simulink model "VCU_CS75_12_16_Test"  (R2014a)
settings: Solver=FixedStepDiscrete  StartTime=0.0  StopTime=25  FixedStep=0.0005  RelTol=1e-3
undefined symbols (not defined in the file): ecucoder_acal, I_SW01_L, LaterlAngleCommand, LDW, RemoteAcclPosition
libraries: simulink x913, ec5744lib x39
(part 6 of 30)

== system VCU_CS75_12_16_Test/长安CS75底盘程序，20ms一次/Input/DBC转化的messages（存底）/ReceiveMessages18/BCM_328 ==
  input : Inport
  Demux : Demux  Outputs=8
  LCM_DRLSts_Ad : Sum
  LCM_DRLSts_Convert : DataTypeConversion  OutDataTypeStr=uint32
  LCM_DRLSts_F : Gain
  LCM_DRLSts_L : simulink/Logic and Bit Operations/Bitwise Operator  logicop=AND  UseBitMask=on  BitMask=192  BitMaskRealWorld=Stored Integer
  LCM_DRLSts_O : Constant  Value=0  OutDataTypeStr=single
  LCM_DRLSts_S : ArithShift  BitShiftNumber=6
  LCM_DRLSts_Sub : Subsystem
  LCM_DRLSts_sat : Saturate  UpperLimit=0  LowerLimit=0
  LCM_DRLStscv : DataTypeConversion
  LCM_DriveMode_Ad : Sum
  LCM_DriveMode_Convert : DataTypeConversion  OutDataTypeStr=uint32
  LCM_DriveMode_F : Gain
  LCM_DriveMode_L : simulink/Logic and Bit Operations/Bitwise Operator  logicop=AND  UseBitMask=on  BitMask=192  BitMaskRealWorld=Stored Integer
  LCM_DriveMode_O : Constant  Value=0  OutDataTypeStr=single
  LCM_DriveMode_S : ArithShift  BitShiftNumber=6
  LCM_DriveMode_Sub : Subsystem
  LCM_DriveMode_sat : Saturate  UpperLimit=0  LowerLimit=0
  LCM_DriveModecv : DataTypeConversion
  LCM_LASSwitch_Ad : Sum
  LCM_LASSwitch_Convert : DataTypeConversion  OutDataTypeStr=uint32
  LCM_LASSwitch_F : Gain
  LCM_LASSwitch_L : simulink/Logic and Bit Operations/Bitwise Operator  logicop=AND  UseBitMask=on  BitMask=3  BitMaskRealWorld=Stored Integer
  LCM_LASSwitch_O : Constant  Value=0  OutDataTypeStr=single
  LCM_LASSwitch_S : ArithShift
  LCM_LASSwitch_Sub : Subsystem
  LCM_LASSwitch_sat : Saturate  UpperLimit=3  LowerLimit=0
  LCM_LASSwitchcv : DataTypeConversion
  LCM_RearLeftTuningLightFaultSts_Ad : Sum
  LCM_RearLeftTuningLightFaultSts_Convert : DataTypeConversion  OutDataTypeStr=uint32
  LCM_RearLeftTuningLightFaultSts_F : Gain
  LCM_RearLeftTuningLightFaultSts_L : simulink/Logic and Bit Operations/Bitwise Operator  logicop=AND  UseBitMask=on  BitMask=128  BitMaskRealWorld=Stored Integer
  LCM_RearLeftTuningLightFaultSts_O : Constant  Value=0  OutDataTypeStr=single
  LCM_RearLeftTuningLightFaultSts_S : ArithShift  BitShiftNumber=7
  LCM_RearLeftTuningLightFaultSts_Sub : Subsystem
  LCM_RearLeftTuningLightFaultSts_sat : Saturate  UpperLimit=0  LowerLimit=0
  LCM_RearLeftTuningLightFaultStscv : DataTypeConversion
  LCM_RearRightTuningLightFaultSts_Ad : Sum
  LCM_RearRightTuningLightFaultSts_Convert : DataTypeConversion  OutDataTypeStr=uint32
  LCM_RearRightTuningLightFaultSts_F : Gain
  LCM_RearRightTuningLightFaultSts_L : simulink/Logic and Bit Operations/Bitwise Operator  logicop=AND  UseBitMask=on  BitMask=128  BitMaskRealWorld=Stored Integer
  LCM_RearRightTuningLightFaultSts_O : Constant  Value=0  OutDataTypeStr=single
  LCM_RearRightTuningLightFaultSts_S : ArithShift  BitShiftNumber=7
  LCM_RearRightTuningLightFaultSts_Sub : Subsystem
  LCM_RearRightTuningLightFaultSts_sat : Saturate  UpperLimit=0  LowerLimit=0
  LCM_RearRightTuningLightFaultStscv : DataTypeConversion
  LCM_ReverseLightSts_Ad : Sum
  LCM_ReverseLightSts_Convert : DataTypeConversion  OutDataTypeStr=uint32
  LCM_ReverseLightSts_F : Gain
  LCM_ReverseLightSts_L : simulink/Logic and Bit Operations/Bitwise Operator  logicop=AND  UseBitMask=on  BitMask=192  BitMaskRealWorld=Stored Integer
  LCM_ReverseLightSts_O : Constant  Value=0  OutDataTypeStr=single
  LCM_ReverseLightSts_S : ArithShift  BitShiftNumber=6
  LCM_ReverseLightSts_Sub : Subsystem
  LCM_ReverseLightSts_sat : Saturate  UpperLimit=0  LowerLimit=0
  LCM_ReverseLightStscv : DataTypeConversion
  LCM_DriveMode_Out : Outport
  LCM_DRLSts_Out : Outport  Port=2
  LCM_LASSwitch_Out : Outport  Port=3
  LCM_RearRightTuningLightFaultSts_Out : Outport  Port=4
  LCM_RearLeftTuningLightFaultSts_Out : Outport  Port=5
  LCM_ReverseLightSts_Out : Outport  Port=6
  wires:
  input/1 -> Demux/1
  LCM_ReverseLightStscv/1 -> LCM_ReverseLightSts_F/1
  LCM_ReverseLightSts_S/1 -> LCM_ReverseLightStscv/1
  LCM_ReverseLightSts_L/1 -> LCM_ReverseLightSts_S/1
  LCM_ReverseLightSts_Convert/1 -> LCM_ReverseLightSts_L/1
  LCM_ReverseLightSts_Sub/1(Out1) -> LCM_ReverseLightSts_Convert/1
  Demux/6 -> LCM_ReverseLightSts_Sub/1(In1)
  LCM_ReverseLightSts_sat/1 -> LCM_ReverseLightSts_Out/1
  LCM_ReverseLightSts_Ad/1 -> LCM_ReverseLightSts_sat/1
  LCM_ReverseLightSts_O/1 -> LCM_ReverseLightSts_Ad/2
  LCM_ReverseLightSts_F/1 -> LCM_ReverseLightSts_Ad/1
  LCM_RearLeftTuningLightFaultStscv/1 -> LCM_RearLeftTuningLightFaultSts_F/1
  LCM_RearLeftTuningLightFaultSts_S/1 -> LCM_RearLeftTuningLightFaultStscv/1
  LCM_RearLeftTuningLightFaultSts_L/1 -> LCM_RearLeftTuningLightFaultSts_S/1
  LCM_RearLeftTuningLightFaultSts_Convert/1 -> LCM_RearLeftTuningLightFaultSts_L/1
  LCM_RearLeftTuningLightFaultSts_Sub/1(Out1) -> LCM_RearLeftTuningLightFaultSts_Convert/1
  Demux/5 -> LCM_RearLeftTuningLightFaultSts_Sub/1(In1)
  LCM_RearLeftTuningLightFaultSts_sat/1 -> LCM_RearLeftTuningLightFaultSts_Out/1
  LCM_RearLeftTuningLightFaultSts_Ad/1 -> LCM_RearLeftTuningLightFaultSts_sat/1
  LCM_RearLeftTuningLightFaultSts_O/1 -> LCM_RearLeftTuningLightFaultSts_Ad/2
  LCM_RearLeftTuningLightFaultSts_F/1 -> LCM_RearLeftTuningLightFaultSts_Ad/1
  LCM_RearRightTuningLightFaultStscv/1 -> LCM_RearRightTuningLightFaultSts_F/1
  LCM_RearRightTuningLightFaultSts_S/1 -> LCM_RearRightTuningLightFaultStscv/1
  LCM_RearRightTuningLightFaultSts_L/1 -> LCM_RearRightTuningLightFaultSts_S/1
  LCM_RearRightTuningLightFaultSts_Convert/1 -> LCM_RearRightTuningLightFaultSts_L/1
  LCM_RearRightTuningLightFaultSts_Sub/1(Out1) -> LCM_RearRightTuningLightFaultSts_Convert/1
  Demux/4 -> LCM_RearRightTuningLightFaultSts_Sub/1(In1)
  LCM_RearRightTuningLightFaultSts_sat/1 -> LCM_RearRightTuningLightFaultSts_Out/1
  LCM_RearRightTuningLightFaultSts_Ad/1 -> LCM_RearRightTuningLightFaultSts_sat/1
  LCM_RearRightTuningLightFaultSts_O/1 -> LCM_RearRightTuningLightFaultSts_Ad/2
  LCM_RearRightTuningLightFaultSts_F/1 -> LCM_RearRightTuningLightFaultSts_Ad/1
  LCM_LASSwitchcv/1 -> LCM_LASSwitch_F/1
  LCM_LASSwitch_S/1 -> LCM_LASSwitchcv/1
  LCM_LASSwitch_L/1 -> LCM_LASSwitch_S/1
  LCM_LASSwitch_Convert/1 -> LCM_LASSwitch_L/1
  LCM_LASSwitch_Sub/1(Out1) -> LCM_LASSwitch_Convert/1
  Demux/3 -> LCM_LASSwitch_Sub/1(In1)
  LCM_LASSwitch_sat/1 -> LCM_LASSwitch_Out/1
  LCM_LASSwitch_Ad/1 -> LCM_LASSwitch_sat/1
  LCM_LASSwitch_O/1 -> LCM_LASSwitch_Ad/2
  LCM_LASSwitch_F/1 -> LCM_LASSwitch_Ad/1
  LCM_DRLStscv/1 -> LCM_DRLSts_F/1
  LCM_DRLSts_S/1 -> LCM_DRLStscv/1
  LCM_DRLSts_L/1 -> LCM_DRLSts_S/1
  LCM_DRLSts_Convert/1 -> LCM_DRLSts_L/1
  LCM_DRLSts_Sub/1(Out1) -> LCM_DRLSts_Convert/1
  Demux/2 -> LCM_DRLSts_Sub/1(In1)
  LCM_DRLSts_sat/1 -> LCM_DRLSts_Out/1
  LCM_DRLSts_Ad/1 -> LCM_DRLSts_sat/1
  LCM_DRLSts_O/1 -> LCM_DRLSts_Ad/2
  LCM_DRLSts_F/1 -> LCM_DRLSts_Ad/1
  LCM_DriveModecv/1 -> LCM_DriveMode_F/1
  LCM_DriveMode_S/1 -> LCM_DriveModecv/1
  LCM_DriveMode_L/1 -> LCM_DriveMode_S/1
  LCM_DriveMode_Convert/1 -> LCM_DriveMode_L/1
  LCM_DriveMode_Sub/1(Out1) -> LCM_DriveMode_Convert/1
  Demux/1 -> LCM_DriveMode_Sub/1(In1)
  LCM_DriveMode_sat/1 -> LCM_DriveMode_Out/1
  LCM_DriveMode_Ad/1 -> LCM_DriveMode_sat/1
  LCM_DriveMode_O/1 -> LCM_DriveMode_Ad/2
  LCM_DriveMode_F/1 -> LCM_DriveMode_Ad/1

== system VCU_CS75_12_16_Test/长安CS75底盘程序，20ms一次/Input/DBC转化的messages（存底）/ReceiveMessages19/BCM_348 ==
  input : Inport
  BCM_DriveMode_Ad : Sum
  BCM_DriveMode_Convert : DataTypeConversion  OutDataTypeStr=uint32
  BCM_DriveMode_F : Gain
  BCM_DriveMode_L : simulink/Logic and Bit Operations/Bitwise Operator  logicop=AND  UseBitMask=on  BitMask=6  BitMaskRealWorld=Stored Integer
  BCM_DriveMode_O : Constant  Value=0  OutDataTypeStr=single
  BCM_DriveMode_S : ArithShift  BitShiftNumber=1
  BCM_DriveMode_Sub : Subsystem
  BCM_DriveMode_sat : Saturate  UpperLimit=3  LowerLimit=0
  BCM_DriveModecv : DataTypeConversion
  BCM_LockSignal_Ad : Sum
  BCM_LockSignal_Convert : DataTypeConversion  OutDataTypeStr=uint32
  BCM_LockSignal_F : Gain
  BCM_LockSignal_L : simulink/Logic and Bit Operations/Bitwise Operator  logicop=AND  UseBitMask=on  BitMask=24  BitMaskRealWorld=Stored Integer
  BCM_LockSignal_O : Constant  Value=0  OutDataTypeStr=single
  BCM_LockSignal_S : ArithShift  BitShiftNumber=3
  BCM_LockSignal_Sub : Subsystem
  BCM_LockSignal_sat : Saturate  UpperLimit=3  LowerLimit=0
  BCM_LockSignalcv : DataTypeConversion
  BCM_UnlockSignal_Ad : Sum
  BCM_UnlockSignal_Convert : DataTypeConversion  OutDataTypeStr=uint32
  BCM_UnlockSignal_F : Gain
  BCM_UnlockSignal_L : simulink/Logic and Bit Operations/Bitwise Operator  logicop=AND  UseBitMask=on  BitMask=96  BitMaskRealWorld=Stored Integer
  BCM_UnlockSignal_O : Constant  Value=0  OutDataTypeStr=single
  BCM_UnlockSignal_S : ArithShift  BitShiftNumber=5
  BCM_UnlockSignal_Sub : Subsystem
  BCM_UnlockSignal_sat : Saturate  UpperLimit=3  LowerLimit=0
  BCM_UnlockSignalcv : DataTypeConversion
  Demux : Demux  Outputs=8
  BCM_DriveMode_Out : Outport
  BCM_LockSignal_Out : Outport  Port=2
  BCM_UnlockSignal_Out : Outport  Port=3
  wires:
  input/1 -> Demux/1
  BCM_UnlockSignalcv/1 -> BCM_UnlockSignal_F/1
  BCM_UnlockSignal_S/1 -> BCM_UnlockSignalcv/1
  BCM_UnlockSignal_L/1 -> BCM_UnlockSignal_S/1
  BCM_UnlockSignal_Convert/1 -> BCM_UnlockSignal_L/1
  BCM_UnlockSignal_Sub/1(Out1) -> BCM_UnlockSignal_Convert/1
  BCM_UnlockSignal_sat/1 -> BCM_UnlockSignal_Out/1
  BCM_UnlockSignal_Ad/1 -> BCM_UnlockSignal_sat/1
  BCM_UnlockSignal_O/1 -> BCM_UnlockSignal_Ad/2
  BCM_UnlockSignal_F/1 -> BCM_UnlockSignal_Ad/1
  BCM_LockSignalcv/1 -> BCM_LockSignal_F/1
  BCM_LockSignal_S/1 -> BCM_LockSignalcv/1
  BCM_LockSignal_L/1 -> BCM_LockSignal_S/1
  BCM_LockSignal_Convert/1 -> BCM_LockSignal_L/1
  BCM_LockSignal_Sub/1(Out1) -> BCM_LockSignal_Convert/1
  BCM_LockSignal_sat/1 -> BCM_LockSignal_Out/1
  BCM_LockSignal_Ad/1 -> BCM_LockSignal_sat/1
  BCM_LockSignal_O/1 -> BCM_LockSignal_Ad/2
  BCM_LockSignal_F/1 -> BCM_LockSignal_Ad/1
  BCM_DriveModecv/1 -> BCM_DriveMode_F/1
  BCM_DriveMode_S/1 -> BCM_DriveModecv/1
  BCM_DriveMode_L/1 -> BCM_DriveMode_S/1
  BCM_DriveMode_Convert/1 -> BCM_DriveMode_L/1
  BCM_DriveMode_Sub/1(Out1) -> BCM_DriveMode_Convert/1
  Demux/6 -> BCM_UnlockSignal_Sub/1(In1), BCM_LockSignal_Sub/1(In1), BCM_DriveMode_Sub/1(In1)
  BCM_DriveMode_sat/1 -> BCM_DriveMode_Out/1
  BCM_DriveMode_Ad/1 -> BCM_DriveMode_sat/1
  BCM_DriveMode_O/1 -> BCM_DriveMode_Ad/2
  BCM_DriveMode_F/1 -> BCM_DriveMode_Ad/1

== system VCU_CS75_12_16_Test/长安CS75底盘程序，20ms一次/Input/DBC转化的messages（存底）/ReceiveMessages2/EMS_265 ==
  input : Inport
  Demux : Demux  Outputs=8
  EMS_EngineStatus_Ad : Sum
  EMS_EngineStatus_Convert : DataTypeConversion  OutDataTypeStr=uint32
  EMS_EngineStatus_F : Gain
  EMS_EngineStatus_L : simulink/Logic and Bit Operations/Bitwise Operator  logicop=AND  UseBitMask=on  BitMask=192  BitMaskRealWorld=Stored Integer
  EMS_EngineStatus_O : Constant  Value=0  OutDataTypeStr=single
  EMS_EngineStatus_S : ArithShift  BitShiftNumber=6
  EMS_EngineStatus_Sub : Subsystem
  EMS_EngineStatus_sat : Saturate  UpperLimit=3  LowerLimit=0
  EMS_EngineStatuscv : DataTypeConversion
  EMS_FullLoadIndicatedTorq_Ad : Sum
  EMS_FullLoadIndicatedTorq_Convert : DataTypeConversion  OutDataTypeStr=uint32
  EMS_FullLoadIndicatedTorq_F : Gain  Gain=0.392
  EMS_FullLoadIndicatedTorq_L : simulink/Logic and Bit Operations/Bitwise Operator  logicop=AND  UseBitMask=on  BitMask=255  BitMaskRealWorld=Stored Integer
  EMS_FullLoadIndicatedTorq_O : Constant  Value=0  OutDataTypeStr=single
  EMS_FullLoadIndicatedTorq_S : ArithShift
  EMS_FullLoadIndicatedTorq_Sub : Subsystem
  EMS_FullLoadIndicatedTorq_sat : Saturate  UpperLimit=99.96  LowerLimit=0
  EMS_FullLoadIndicatedTorqcv : DataTypeConversion
  EMS_RollingCounter_id265_Ad : Sum
  EMS_RollingCounter_id265_Convert : DataTypeConversion  OutDataTypeStr=uint32
  EMS_RollingCounter_id265_F : Gain
  EMS_RollingCounter_id265_L : simulink/Logic and Bit Operations/Bitwise Operator  logicop=AND  UseBitMask=on  BitMask=15  BitMaskRealWorld=Stored Integer
  EMS_RollingCounter_id265_O : Constant  Value=0  OutDataTypeStr=single
  EMS_RollingCounter_id265_S : ArithShift
  EMS_RollingCounter_id265_Sub : Subsystem
  EMS_RollingCounter_id265_sat : Saturate  UpperLimit=15  LowerLimit=0
  EMS_RollingCounter_id265cv : DataTypeConversion
  EMS_TorqueConstant_Ad : Sum
  EMS_TorqueConstant_Convert : DataTypeConversion  OutDataTypeStr=uint32
  EMS_TorqueConstant_F : Gain  Gain=10
  EMS_TorqueConstant_L : simulink/Logic and Bit Operations/Bitwise Operator  logicop=AND  UseBitMask=on  BitMask=255  BitMaskRealWorld=Stored Integer
  EMS_TorqueConstant_O : Constant  Value=0  OutDataTypeStr=single
  EMS_TorqueConstant_S : ArithShift
  EMS_TorqueConstant_Sub : Subsystem
  EMS_TorqueConstant_sat : Saturate  UpperLimit=2540  LowerLimit=0
  EMS_TorqueConstantcv : DataTypeConversion
  EMS_FullLoadIndicatedTorq_Out : Outport
  EMS_TorqueConstant_Out : Outport  Port=2
  EMS_RollingCounter_id265_Out : Outport  Port=3
  EMS_EngineStatus_Out : Outport  Port=4
  wires:
  EMS_FullLoadIndicatedTorq_F/1 -> EMS_FullLoadIndicatedTorq_Ad/1
  EMS_FullLoadIndicatedTorq_O/1 -> EMS_FullLoadIndicatedTorq_Ad/2
  EMS_FullLoadIndicatedTorq_Ad/1 -> EMS_FullLoadIndicatedTorq_sat/1
  EMS_FullLoadIndicatedTorq_sat/1 -> EMS_FullLoadIndicatedTorq_Out/1
  Demux/3 -> EMS_FullLoadIndicatedTorq_Sub/1(In1)
  EMS_FullLoadIndicatedTorq_Sub/1(Out1) -> EMS_FullLoadIndicatedTorq_Convert/1
  EMS_FullLoadIndicatedTorq_Convert/1 -> EMS_FullLoadIndicatedTorq_L/1
  EMS_FullLoadIndicatedTorq_L/1 -> EMS_FullLoadIndicatedTorq_S/1
  EMS_FullLoadIndicatedTorq_S/1 -> EMS_FullLoadIndicatedTorqcv/1
  EMS_FullLoadIndicatedTorqcv/1 -> EMS_FullLoadIndicatedTorq_F/1
  EMS_TorqueConstant_F/1 -> EMS_TorqueConstant_Ad/1
  EMS_TorqueConstant_O/1 -> EMS_TorqueConstant_Ad/2
  EMS_TorqueConstant_Ad/1 -> EMS_TorqueConstant_sat/1
  EMS_TorqueConstant_sat/1 -> EMS_TorqueConstant_Out/1
  Demux/7 -> EMS_TorqueConstant_Sub/1(In1)
  EMS_TorqueConstant_Sub/1(Out1) -> EMS_TorqueConstant_Convert/1
  EMS_TorqueConstant_Convert/1 -> EMS_TorqueConstant_L/1
  EMS_TorqueConstant_L/1 -> EMS_TorqueConstant_S/1
  EMS_TorqueConstant_S/1 -> EMS_TorqueConstantcv/1
  EMS_TorqueConstantcv/1 -> EMS_TorqueConstant_F/1
  EMS_RollingCounter_id265_F/1 -> EMS_RollingCounter_id265_Ad/1
  EMS_RollingCounter_id265_O/1 -> EMS_RollingCounter_id265_Ad/2
  EMS_RollingCounter_id265_Ad/1 -> EMS_RollingCounter_id265_sat/1
  EMS_RollingCounter_id265_sat/1 -> EMS_RollingCounter_id265_Out/1
  Demux/8 -> EMS_RollingCounter_id265_Sub/1(In1), EMS_EngineStatus_Sub/1(In1)
  EMS_RollingCounter_id265_Sub/1(Out1) -> EMS_RollingCounter_id265_Convert/1
  EMS_RollingCounter_id265_Convert/1 -> EMS_RollingCounter_id265_L/1
  EMS_RollingCounter_id265_L/1 -> EMS_RollingCounter_id265_S/1
  EMS_RollingCounter_id265_S/1 -> EMS_RollingCounter_id265cv/1
  EMS_RollingCounter_id265cv/1 -> EMS_RollingCounter_id265_F/1
  EMS_EngineStatus_F/1 -> EMS_EngineStatus_Ad/1
  EMS_EngineStatus_O/1 -> EMS_EngineStatus_Ad/2
  EMS_EngineStatus_Ad/1 -> EMS_EngineStatus_sat/1
  EMS_EngineStatus_sat/1 -> EMS_EngineStatus_Out/1
  EMS_EngineStatus_Sub/1(Out1) -> EMS_EngineStatus_Convert/1
  EMS_EngineStatus_Convert/1 -> EMS_EngineStatus_L/1
  EMS_EngineStatus_L/1 -> EMS_EngineStatus_S/1
  EMS_EngineStatus_S/1 -> EMS_EngineStatuscv/1
  EMS_EngineStatuscv/1 -> EMS_EngineStatus_F/1
  input/1 -> Demux/1

== system VCU_CS75_12_16_Test/长安CS75底盘程序，20ms一次/Input/DBC转化的messages（存底）/ReceiveMessages20/BCM_3DF ==
  input : Inport
  BCM_AmbientLightColorFeedback_Ad : Sum
  BCM_AmbientLightColorFeedback_Convert : DataTypeConversion  OutDataTypeStr=uint32
  BCM_AmbientLightColorFeedback_F : Gain
  BCM_AmbientLightColorFeedback_L : simulink/Logic and Bit Operations/Bitwise Operator  logicop=AND  UseBitMask=on  BitMask=255  BitMaskRealWorld=Stored Integer
  BCM_AmbientLightColorFeedback_O : Constant  Value=0  OutDataTypeStr=single
  BCM_AmbientLightColorFeedback_S : ArithShift
  BCM_AmbientLightColorFeedback_Sub : Subsystem
  BCM_AmbientLightColorFeedback_sat : Saturate  UpperLimit=255  LowerLimit=0
  BCM_AmbientLightColorFeedbackcv : DataTypeConversion
  BCM_CRC_Checksum_Ad : Sum
  BCM_CRC_Checksum_Convert : DataTypeConversion  OutDataTypeStr=uint32
  BCM_CRC_Checksum_F : Gain
  BCM_CRC_Checksum_L : simulink/Logic and Bit Operations/Bitwise Operator  logicop=AND  UseBitMask=on  BitMask=255  BitMaskRealWorld=Stored Integer
  BCM_CRC_Checksum_O : Constant  Value=0  OutDataTypeStr=single
  BCM_CRC_Checksum_S : ArithShift
  BCM_CRC_Checksum_Sub : Subsystem
  BCM_CRC_Checksum_sat : Saturate  UpperLimit=0  LowerLimit=0
  BCM_CRC_Checksumcv : DataTypeConversion
  BCM_DriveModeFeedback_Ad : Sum
  BCM_DriveModeFeedback_Convert : DataTypeConversion  OutDataTypeStr=uint32
  BCM_DriveModeFeedback_F : Gain
  BCM_DriveModeFeedback_L : simulink/Logic and Bit Operations/Bitwise Operator  logicop=AND  UseBitMask=on  BitMask=48  BitMaskRealWorld=Stored Integer
  BCM_DriveModeFeedback_O : Constant  Value=0  OutDataTypeStr=single
  BCM_DriveModeFeedback_S : ArithShift  BitShiftNumber=4
  BCM_DriveModeFeedback_Sub : Subsystem
  BCM_DriveModeFeedback_sat : Saturate  UpperLimit=3  LowerLimit=0
  BCM_DriveModeFeedbackcv : DataTypeConversion
  BCM_DriveModeStatus_Ad : Sum
  BCM_DriveModeStatus_Convert : DataTypeConversion  OutDataTypeStr=uint32
  BCM_DriveModeStatus_F : Gain
  BCM_DriveModeStatus_L : simulink/Logic and Bit Operations/Bitwise Operator  logicop=AND  UseBitMask=on  BitMask=15  BitMaskRealWorld=Stored Integer
  BCM_DriveModeStatus_O : Constant  Value=0  OutDataTypeStr=single
  BCM_DriveModeStatus_S : ArithShift
  BCM_DriveModeStatus_Sub : Subsystem
  BCM_DriveModeStatus_sat : Saturate  UpperLimit=15  LowerLimit=0
  BCM_DriveModeStatuscv : DataTypeConversion
  BCM_DriveMode_Ad : Sum
  BCM_DriveMode_Convert : DataTypeConversion  OutDataTypeStr=uint32
  BCM_DriveMode_F : Gain
  BCM_DriveMode_L : simulink/Logic and Bit Operations/Bitwise Operator  logicop=AND  UseBitMask=on  BitMask=240  BitMaskRealWorld=Stored Integer
  BCM_DriveMode_O : Constant  Value=0  OutDataTypeStr=single
  BCM_DriveMode_S : ArithShift  BitShiftNumber=4
  BCM_DriveMode_Sub : Subsystem
  BCM_DriveMode_sat : Saturate  UpperLimit=0  LowerLimit=0
  BCM_DriveModecv : DataTypeConversion
  BCM_EPSTorqueModeFeedback_Ad : Sum
  BCM_EPSTorqueModeFeedback_Convert : DataTypeConversion  OutDataTypeStr=uint32
  BCM_EPSTorqueModeFeedback_F : Gain
  BCM_EPSTorqueModeFeedback_L : simulink/Logic and Bit Operations/Bitwise Operator  logicop=AND  UseBitMask=on  BitMask=192  BitMaskRealWorld=Stored Integer
  BCM_EPSTorqueModeFeedback_O : Constant  Value=0  OutDataTypeStr=single
  BCM_EPSTorqueModeFeedback_S : ArithShift  BitShiftNumber=6
  BCM_EPSTorqueModeFeedback_Sub : Subsystem
  BCM_EPSTorqueModeFeedback_sat : Saturate  UpperLimit=3  LowerLimit=0
  BCM_EPSTorqueModeFeedbackcv : DataTypeConversion
  BCM_EPSTorqueMode_Ad : Sum
  BCM_EPSTorqueMode_Convert : DataTypeConversion  OutDataTypeStr=uint32
  BCM_EPSTorqueMode_F : Gain
  BCM_EPSTorqueMode_L : simulink/Logic and Bit Operations/Bitwise Operator  logicop=AND  UseBitMask=on  BitMask=6  BitMaskRealWorld=Stored Integer
  BCM_EPSTorqueMode_O : Constant  Value=0  OutDataTypeStr=single
  BCM_EPSTorqueMode_S : ArithShift  BitShiftNumber=1
  BCM_EPSTorqueMode_Sub : Subsystem
  BCM_EPSTorqueMode_sat : Saturate  UpperLimit=3  LowerLimit=0
  BCM_EPSTorqueModecv : DataTypeConversion
  BCM_RollingCounter_Ad : Sum
  BCM_RollingCounter_Convert : DataTypeConversion  OutDataTypeStr=uint32
  BCM_RollingCounter_F : Gain
  BCM_RollingCounter_L : simulink/Logic and Bit Operations/Bitwise Operator  logicop=AND  UseBitMask=on  BitMask=15  BitMaskRealWorld=Stored Integer
  BCM_RollingCounter_O : Constant  Value=0  OutDataTypeStr=single
  BCM_RollingCounter_S : ArithShift
  BCM_RollingCounter_Sub : Subsystem
  BCM_RollingCounter_sat : Saturate  UpperLimit=0  LowerLimit=0
  BCM_RollingCountercv : DataTypeConversion
  Demux : Demux  Outputs=8
  BCM_DriveMode_Out : Outport
  BCM_EPSTorqueMode_Out : Outport  Port=2
  BCM_DriveModeStatus_Out : Outport  Port=3
  BCM_DriveModeFeedback_Out : Outport  Port=4
  BCM_EPSTorqueModeFeedback_Out : Outport  Port=5
  BCM_AmbientLightColorFeedback_Out : Outport  Port=6
  BCM_RollingCounter_Out : Outport  Port=7
  BCM_CRC_Checksum_Out : Outport  Port=8
  wires:
  input/1 -> Demux/1
  BCM_CRC_Checksumcv/1 -> BCM_CRC_Checksum_F/1
  BCM_CRC_Checksum_S/1 -> BCM_CRC_Checksumcv/1
  BCM_CRC_Checksum_L/1 -> BCM_CRC_Checksum_S/1
  BCM_CRC_Checksum_Convert/1 -> BCM_CRC_Checksum_L/1
  BCM_CRC_Checksum_Sub/1(Out1) -> BCM_CRC_Checksum_Convert/1
  Demux/8 -> BCM_CRC_Checksum_Sub/1(In1)
  BCM_CRC_Checksum_sat/1 -> BCM_CRC_Checksum_Out/1
  BCM_CRC_Checksum_Ad/1 -> BCM_CRC_Checksum_sat/1
  BCM_CRC_Checksum_O/1 -> BCM_CRC_Checksum_Ad/2
  BCM_CRC_Checksum_F/1 -> BCM_CRC_Checksum_Ad/1
  BCM_RollingCountercv/1 -> BCM_RollingCounter_F/1
  BCM_RollingCounter_S/1 -> BCM_RollingCountercv/1
  BCM_RollingCounter_L/1 -> BCM_RollingCounter_S/1
  BCM_RollingCounter_Convert/1 -> BCM_RollingCounter_L/1
  BCM_RollingCounter_Sub/1(Out1) -> BCM_RollingCounter_Convert/1
  Demux/7 -> BCM_RollingCounter_Sub/1(In1)
  BCM_RollingCounter_sat/1 -> BCM_RollingCounter_Out/1
  BCM_RollingCounter_Ad/1 -> BCM_RollingCounter_sat/1
  BCM_RollingCounter_O/1 -> BCM_RollingCounter_Ad/2
  BCM_RollingCounter_F/1 -> BCM_RollingCounter_Ad/1
  BCM_AmbientLightColorFeedbackcv/1 -> BCM_AmbientLightColorFeedback_F/1
  BCM_AmbientLightColorFeedback_S/1 -> BCM_AmbientLightColorFeedbackcv/1
  BCM_AmbientLightColorFeedback_L/1 -> BCM_AmbientLightColorFeedback_S/1
  BCM_AmbientLightColorFeedback_Convert/1 -> BCM_AmbientLightColorFeedback_L/1
  BCM_AmbientLightColorFeedback_Sub/1(Out1) -> BCM_AmbientLightColorFeedback_Convert/1
  Demux/4 -> BCM_AmbientLightColorFeedback_Sub/1(In1)
  BCM_AmbientLightColorFeedback_sat/1 -> BCM_AmbientLightColorFeedback_Out/1
  BCM_AmbientLightColorFeedback_Ad/1 -> BCM_AmbientLightColorFeedback_sat/1
  BCM_AmbientLightColorFeedback_O/1 -> BCM_AmbientLightColorFeedback_Ad/2
  BCM_AmbientLightColorFeedback_F/1 -> BCM_AmbientLightColorFeedback_Ad/1
  BCM_EPSTorqueModeFeedbackcv/1 -> BCM_EPSTorqueModeFeedback_F/1
  BCM_EPSTorqueModeFeedback_S/1 -> BCM_EPSTorqueModeFeedbackcv/1
  BCM_EPSTorqueModeFeedback_L/1 -> BCM_EPSTorqueModeFeedback_S/1
  BCM_EPSTorqueModeFeedback_Convert/1 -> BCM_EPSTorqueModeFeedback_L/1
  BCM_EPSTorqueModeFeedback_Sub/1(Out1) -> BCM_EPSTorqueModeFeedback_Convert/1
  BCM_EPSTorqueModeFeedback_sat/1 -> BCM_EPSTorqueModeFeedback_Out/1
  BCM_EPSTorqueModeFeedback_Ad/1 -> BCM_EPSTorqueModeFeedback_sat/1
  BCM_EPSTorqueModeFeedback_O/1 -> BCM_EPSTorqueModeFeedback_Ad/2
  BCM_EPSTorqueModeFeedback_F/1 -> BCM_EPSTorqueModeFeedback_Ad/1
  BCM_DriveModeFeedbackcv/1 -> BCM_DriveModeFeedback_F/1
  BCM_DriveModeFeedback_S/1 -> BCM_DriveModeFeedbackcv/1
  BCM_DriveModeFeedback_L/1 -> BCM_DriveModeFeedback_S/1
  BCM_DriveModeFeedback_Convert/1 -> BCM_DriveModeFeedback_L/1
  BCM_DriveModeFeedback_Sub/1(Out1) -> BCM_DriveModeFeedback_Convert/1
  BCM_DriveModeFeedback_sat/1 -> BCM_DriveModeFeedback_Out/1
  BCM_DriveModeFeedback_Ad/1 -> BCM_DriveModeFeedback_sat/1
  BCM_DriveModeFeedback_O/1 -> BCM_DriveModeFeedback_Ad/2
  BCM_DriveModeFeedback_F/1 -> BCM_DriveModeFeedback_Ad/1
  BCM_DriveModeStatuscv/1 -> BCM_DriveModeStatus_F/1
  BCM_DriveModeStatus_S/1 -> BCM_DriveModeStatuscv/1
  BCM_DriveModeStatus_L/1 -> BCM_DriveModeStatus_S/1
  BCM_DriveModeStatus_Convert/1 -> BCM_DriveModeStatus_L/1
  BCM_DriveModeStatus_Sub/1(Out1) -> BCM_DriveModeStatus_Convert/1
  Demux/3 -> BCM_EPSTorqueModeFeedback_Sub/1(In1), BCM_DriveModeFeedback_Sub/1(In1), BCM_DriveModeStatus_Sub/1(In1)
  BCM_DriveModeStatus_sat/1 -> BCM_DriveModeStatus_Out/1
  BCM_DriveModeStatus_Ad/1 -> BCM_DriveModeStatus_sat/1
  BCM_DriveModeStatus_O/1 -> BCM_DriveModeStatus_Ad/2
  BCM_DriveModeStatus_F/1 -> BCM_DriveModeStatus_Ad/1
  BCM_EPSTorqueModecv/1 -> BCM_EPSTorqueMode_F/1
  BCM_EPSTorqueMode_S/1 -> BCM_EPSTorqueModecv/1
  BCM_EPSTorqueMode_L/1 -> BCM_EPSTorqueMode_S/1
  BCM_EPSTorqueMode_Convert/1 -> BCM_EPSTorqueMode_L/1
  BCM_EPSTorqueMode_Sub/1(Out1) -> BCM_EPSTorqueMode_Convert/1
  Demux/2 -> BCM_EPSTorqueMode_Sub/1(In1)
  BCM_EPSTorqueMode_sat/1 -> BCM_EPSTorqueMode_Out/1
  BCM_EPSTorqueMode_Ad/1 -> BCM_EPSTorqueMode_sat/1
  BCM_EPSTorqueMode_O/1 -> BCM_EPSTorqueMode_Ad/2
  BCM_EPSTorqueMode_F/1 -> BCM_EPSTorqueMode_Ad/1
  BCM_DriveModecv/1 -> BCM_DriveMode_F/1
  BCM_DriveMode_S/1 -> BCM_DriveModecv/1
  BCM_DriveMode_L/1 -> BCM_DriveMode_S/1
  BCM_DriveMode_Convert/1 -> BCM_DriveMode_L/1
  BCM_DriveMode_Sub/1(Out1) -> BCM_DriveMode_Convert/1
  Demux/1 -> BCM_DriveMode_Sub/1(In1)
  BCM_DriveMode_sat/1 -> BCM_DriveMode_Out/1
  BCM_DriveMode_Ad/1 -> BCM_DriveMode_sat/1
  BCM_DriveMode_O/1 -> BCM_DriveMode_Ad/2
  BCM_DriveMode_F/1 -> BCM_DriveMode_Ad/1

== system VCU_CS75_12_16_Test/长安CS75底盘程序，20ms一次/Input/DBC转化的messages（存底）/ReceiveMessages21/GW_20B ==
  input : Inport
  Demux : Demux  Outputs=8
  EMS_BrakePedalStatus_Ad : Sum
  EMS_BrakePedalStatus_Convert : DataTypeConversion  OutDataTypeStr=uint32
  EMS_BrakePedalStatus_F : Gain
  EMS_BrakePedalStatus_L : simulink/Logic and Bit Operations/Bitwise Operator  logicop=AND  UseBitMask=on  BitMask=192  BitMaskRealWorld=Stored Integer
  EMS_BrakePedalStatus_O : Constant  Value=0  OutDataTypeStr=single
  EMS_BrakePedalStatus_S : ArithShift  BitShiftNumber=6
  EMS_BrakePedalStatus_Sub : Subsystem
  EMS_BrakePedalStatus_sat : Saturate  UpperLimit=3  LowerLimit=0
  EMS_BrakePedalStatuscv : DataTypeConversion
  EMS_EngineStartupEnd_Ad : Sum
  EMS_EngineStartupEnd_Convert : DataTypeConversion  OutDataTypeStr=uint32
  EMS_EngineStartupEnd_F : Gain
  EMS_EngineStartupEnd_L : simulink/Logic and Bit Operations/Bitwise Operator  logicop=AND  UseBitMask=on  BitMask=48  BitMaskRealWorld=Stored Integer
  EMS_EngineStartupEnd_O : Constant  Value=0  OutDataTypeStr=single
  EMS_EngineStartupEnd_S : ArithShift  BitShiftNumber=4
  EMS_EngineStartupEnd_Sub : Subsystem
  EMS_EngineStartupEnd_sat : Saturate  UpperLimit=3  LowerLimit=0
  EMS_EngineStartupEndcv : DataTypeConversion
  EMS_EngineStatus_Ad : Sum
  EMS_EngineStatus_Convert : DataTypeConversion  OutDataTypeStr=uint32
  EMS_EngineStatus_F : Gain
  EMS_EngineStatus_L : simulink/Logic and Bit Operations/Bitwise Operator  logicop=AND  UseBitMask=on  BitMask=48  BitMaskRealWorld=Stored Integer
  EMS_EngineStatus_O : Constant  Value=0  OutDataTypeStr=single
  EMS_EngineStatus_S : ArithShift  BitShiftNumber=4
  EMS_EngineStatus_Sub : Subsystem
  EMS_EngineStatus_sat : Saturate  UpperLimit=3  LowerLimit=0
  EMS_EngineStatuscv : DataTypeConversion
  EPB_BrakeLightOnRequest_Ad : Sum
  EPB_BrakeLightOnRequest_Convert : DataTypeConversion  OutDataTypeStr=uint32
  EPB_BrakeLightOnRequest_F : Gain
  EPB_BrakeLightOnRequest_L : simulink/Logic and Bit Operations/Bitwise Operator  logicop=AND  UseBitMask=on  BitMask=6  BitMaskRealWorld=Stored Integer
  EPB_BrakeLightOnRequest_O : Constant  Value=0  OutDataTypeStr=single
  EPB_BrakeLightOnRequest_S : ArithShift  BitShiftNumber=1
  EPB_BrakeLightOnRequest_Sub : Subsystem
  EPB_BrakeLightOnRequest_sat : Saturate  UpperLimit=3  LowerLimit=0
  EPB_BrakeLightOnRequestcv : DataTypeConversion
  EPB_Status_Ad : Sum
  EPB_Status_Convert : DataTypeConversion  OutDataTypeStr=uint32
  EPB_Status_F : Gain
  EPB_Status_L : simulink/Logic and Bit Operations/Bitwise Operator  logicop=AND  UseBitMask=on  BitMask=192  BitMaskRealWorld=Stored Integer
  EPB_Status_O : Constant  Value=0  OutDataTypeStr=single
  EPB_Status_S : ArithShift  BitShiftNumber=6
  EPB_Status_Sub : Subsystem
  EPB_Status_sat : Saturate  UpperLimit=3  LowerLimit=0
  EPB_Statuscv : DataTypeConversion
  SAS_SteeringAngleCS : ArithShift  BitShiftNumber=-16
  SAS_SteeringAngleCS1 : ArithShift  BitShiftNumber=-15
  SAS_SteeringAngleConS : Constant  OutDataTypeStr=single
  SAS_SteeringAngleMinus : UnaryMinus
  SAS_SteeringAngleROP : RelationalOperator  OutDataTypeStr=boolean
  SAS_SteeringAngleSW : Switch  Criteria=u2 ~= 0
  SAS_SteeringAngleValid_Ad : Sum
  SAS_SteeringAngleValid_Convert : DataTypeConversion  OutDataTypeStr=uint32
  SAS_SteeringAngleValid_F : Gain
  SAS_SteeringAngleValid_L : simulink/Logic and Bit Operations/Bitwise Operator  logicop=AND  UseBitMask=on  BitMask=1  BitMaskRealWorld=Stored Integer
  SAS_SteeringAngleValid_O : Constant  Value=0  OutDataTypeStr=single
  SAS_SteeringAngleValid_S : ArithShift
  SAS_SteeringAngleValid_Sub : Subsystem
  SAS_SteeringAngleValid_sat : Saturate  UpperLimit=1  LowerLimit=0
  SAS_SteeringAngleValidcv : DataTypeConversion
  SAS_SteeringAngle_Ad : Sum
  SAS_SteeringAngle_Convert : DataTypeConversion  OutDataTypeStr=uint32
  SAS_SteeringAngle_F : Gain  Gain=0.1
  SAS_SteeringAngle_L : simulink/Logic and Bit Operations/Bitwise Operator  logicop=AND  UseBitMask=on  BitMask=65535  BitMaskRealWorld=Stored Integer
  SAS_SteeringAngle_O : Constant  Value=0  OutDataTypeStr=single
  SAS_SteeringAngle_S : ArithShift
  SAS_SteeringAngle_Sub : Subsystem
  SAS_SteeringAngle_sat : Saturate  UpperLimit=780  LowerLimit=-780
  SAS_SteeringAnglecv : DataTypeConversion
  SAS_SteeringAngleinput4_Ad : Sum
  SAS_SteeringAngleinput4_C : Constant  Value=256
  SAS_SteeringAngleinput4_P : Product
  SAS_SteeringAnglesubcon : Sum  Inputs=+-
  TCU_GearShiftPositon_Ad : Sum
  TCU_GearShiftPositon_Convert : DataTypeConversion  OutDataTypeStr=uint32
  TCU_GearShiftPositon_F : Gain
  TCU_GearShiftPositon_L : simulink/Logic and Bit Operations/Bitwise Operator  logicop=AND  UseBitMask=on  BitMask=120  BitMaskRealWorld=Stored Integer
  TCU_GearShiftPositon_O : Constant  Value=0  OutDataTypeStr=single
  TCU_GearShiftPositon_S : ArithShift  BitShiftNumber=3
  TCU_GearShiftPositon_Sub : Subsystem
  TCU_GearShiftPositon_sat : Saturate  UpperLimit=15  LowerLimit=0
  TCU_GearShiftPositoncv : DataTypeConversion
  TCU_ShiftPostionValid_Ad : Sum
  TCU_ShiftPostionValid_Convert : DataTypeConversion  OutDataTypeStr=uint32
  TCU_ShiftPostionValid_F : Gain
  TCU_ShiftPostionValid_L : simulink/Logic and Bit Operations/Bitwise Operator  logicop=AND  UseBitMask=on  BitMask=128  BitMaskRealWorld=Stored Integer
  TCU_ShiftPostionValid_O : Constant  Value=0  OutDataTypeStr=single
  TCU_ShiftPostionValid_S : ArithShift  BitShiftNumber=7
  TCU_ShiftPostionValid_Sub : Subsystem
  TCU_ShiftPostionValid_sat : Saturate  UpperLimit=1  LowerLimit=0
  TCU_ShiftPostionValidcv : DataTypeConversion
  SAS_SteeringAngleValid_Out : Outport
  EMS_EngineStatus_Out : Outport  Port=2
  EMS_BrakePedalStatus_Out : Outport  Port=3
  EMS_EngineStartupEnd_Out : Outport  Port=4
  SAS_SteeringAngle_Out : Outport  Port=5
  EPB_BrakeLightOnRequest_Out : Outport  Port=6
  TCU_GearShiftPositon_Out : Outport  Port=7
  TCU_ShiftPostionValid_Out : Outport  Port=8
  EPB_Status_Out : Outport  Port=9
  wires:
  input/1 -> Demux/1
  EPB_Statuscv/1 -> EPB_Status_F/1
  EPB_Status_S/1 -> EPB_Statuscv/1
  EPB_Status_L/1 -> EPB_Status_S/1
  EPB_Status_Convert/1 -> EPB_Status_L/1
  EPB_Status_Sub/1(Out1) -> EPB_Status_Convert/1
  Demux/7 -> EPB_Status_Sub/1(In1)
  EPB_Status_sat/1 -> EPB_Status_Out/1
  EPB_Status_Ad/1 -> EPB_Status_sat/1
  EPB_Status_O/1 -> EPB_Status_Ad/2
  EPB_Status_F/1 -> EPB_Status_Ad/1
  TCU_ShiftPostionValidcv/1 -> TCU_ShiftPostionValid_F/1
  TCU_ShiftPostionValid_S/1 -> TCU_ShiftPostionValidcv/1
  TCU_ShiftPostionValid_L/1 -> TCU_ShiftPostionValid_S/1
  TCU_ShiftPostionValid_Convert/1 -> TCU_ShiftPostionValid_L/1
  TCU_ShiftPostionValid_Sub/1(Out1) -> TCU_ShiftPostionValid_Convert/1
  TCU_ShiftPostionValid_sat/1 -> TCU_ShiftPostionValid_Out/1
  TCU_ShiftPostionValid_Ad/1 -> TCU_ShiftPostionValid_sat/1
  TCU_ShiftPostionValid_O/1 -> TCU_ShiftPostionValid_Ad/2
  TCU_ShiftPostionValid_F/1 -> TCU_ShiftPostionValid_Ad/1
  TCU_GearShiftPositoncv/1 -> TCU_GearShiftPositon_F/1
  TCU_GearShiftPositon_S/1 -> TCU_GearShiftPositoncv/1
  TCU_GearShiftPositon_L/1 -> TCU_GearShiftPositon_S/1
  TCU_GearShiftPositon_Convert/1 -> TCU_GearShiftPositon_L/1
  TCU_GearShiftPositon_Sub/1(Out1) -> TCU_GearShiftPositon_Convert/1
  TCU_GearShiftPositon_sat/1 -> TCU_GearShiftPositon_Out/1
  TCU_GearShiftPositon_Ad/1 -> TCU_GearShiftPositon_sat/1
  TCU_GearShiftPositon_O/1 -> TCU_GearShiftPositon_Ad/2
  TCU_GearShiftPositon_F/1 -> TCU_GearShiftPositon_Ad/1
  EPB_BrakeLightOnRequestcv/1 -> EPB_BrakeLightOnRequest_F/1
  EPB_BrakeLightOnRequest_S/1 -> EPB_BrakeLightOnRequestcv/1
  EPB_BrakeLightOnRequest_L/1 -> EPB_BrakeLightOnRequest_S/1
  EPB_BrakeLightOnRequest_Convert/1 -> EPB_BrakeLightOnRequest_L/1
  EPB_BrakeLightOnRequest_Sub/1(Out1) -> EPB_BrakeLightOnRequest_Convert/1
  Demux/6 -> TCU_ShiftPostionValid_Sub/1(In1), TCU_GearShiftPositon_Sub/1(In1), EPB_BrakeLightOnRequest_Sub/1(In1)
  EPB_BrakeLightOnRequest_sat/1 -> EPB_BrakeLightOnRequest_Out/1
  EPB_BrakeLightOnRequest_Ad/1 -> EPB_BrakeLightOnRequest_sat/1
  EPB_BrakeLightOnRequest_O/1 -> EPB_BrakeLightOnRequest_Ad/2
  EPB_BrakeLightOnRequest_F/1 -> EPB_BrakeLightOnRequest_Ad/1
  SAS_SteeringAngleROP/1 -> SAS_SteeringAngleSW/2
  SAS_SteeringAngleSW/1 -> SAS_SteeringAngle_F/1
  SAS_SteeringAngleMinus/1 -> SAS_SteeringAngleSW/1
  SAS_SteeringAnglesubcon/1 -> SAS_SteeringAngleMinus/1
  SAS_SteeringAngleCS/1 -> SAS_SteeringAnglesubcon/1
  SAS_SteeringAngleCS1/1 -> SAS_SteeringAngleROP/2
  SAS_SteeringAngleConS/1 -> SAS_SteeringAngleCS1/1, SAS_SteeringAngleCS/1
  SAS_SteeringAnglecv/1 -> SAS_SteeringAngleSW/3, SAS_SteeringAnglesubcon/2, SAS_SteeringAngleROP/1
  SAS_SteeringAngle_S/1 -> SAS_SteeringAnglecv/1
  SAS_SteeringAngle_L/1 -> SAS_SteeringAngle_S/1
  SAS_SteeringAngle_Convert/1 -> SAS_SteeringAngle_L/1
  SAS_SteeringAngle_Sub/1(Out1) -> SAS_SteeringAngle_Convert/1
  SAS_SteeringAngleinput4_Ad/1 -> SAS_SteeringAngle_Sub/1(In1)
  Demux/5 -> SAS_SteeringAngleinput4_Ad/2
  SAS_SteeringAngleinput4_P/1 -> SAS_SteeringAngleinput4_Ad/1
  SAS_SteeringAngleinput4_C/1 -> SAS_SteeringAngleinput4_P/2
  Demux/4 -> SAS_SteeringAngleinput4_P/1
  SAS_SteeringAngle_sat/1 -> SAS_SteeringAngle_Out/1
  SAS_SteeringAngle_Ad/1 -> SAS_SteeringAngle_sat/1
  SAS_SteeringAngle_O/1 -> SAS_SteeringAngle_Ad/2
  SAS_SteeringAngle_F/1 -> SAS_SteeringAngle_Ad/1
  EMS_EngineStartupEndcv/1 -> EMS_EngineStartupEnd_F/1
  EMS_EngineStartupEnd_S/1 -> EMS_EngineStartupEndcv/1
  EMS_EngineStartupEnd_L/1 -> EMS_EngineStartupEnd_S/1
  EMS_EngineStartupEnd_Convert/1 -> EMS_EngineStartupEnd_L/1
  EMS_EngineStartupEnd_Sub/1(Out1) -> EMS_EngineStartupEnd_Convert/1
  Demux/2 -> EMS_EngineStartupEnd_Sub/1(In1)
  EMS_EngineStartupEnd_sat/1 -> EMS_EngineStartupEnd_Out/1
  EMS_EngineStartupEnd_Ad/1 -> EMS_EngineStartupEnd_sat/1
  EMS_EngineStartupEnd_O/1 -> EMS_EngineStartupEnd_Ad/2
  EMS_EngineStartupEnd_F/1 -> EMS_EngineStartupEnd_Ad/1
  EMS_BrakePedalStatuscv/1 -> EMS_BrakePedalStatus_F/1
  EMS_BrakePedalStatus_S/1 -> EMS_BrakePedalStatuscv/1
  EMS_BrakePedalStatus_L/1 -> EMS_BrakePedalStatus_S/1
  EMS_BrakePedalStatus_Convert/1 -> EMS_BrakePedalStatus_L/1
  EMS_BrakePedalStatus_Sub/1(Out1) -> EMS_BrakePedalStatus_Convert/1
  EMS_BrakePedalStatus_sat/1 -> EMS_BrakePedalStatus_Out/1
  EMS_BrakePedalStatus_Ad/1 -> EMS_BrakePedalStatus_sat/1
  EMS_BrakePedalStatus_O/1 -> EMS_BrakePedalStatus_Ad/2
  EMS_BrakePedalStatus_F/1 -> EMS_BrakePedalStatus_Ad/1
  EMS_EngineStatuscv/1 -> EMS_EngineStatus_F/1
  EMS_EngineStatus_S/1 -> EMS_EngineStatuscv/1
  EMS_EngineStatus_L/1 -> EMS_EngineStatus_S/1
  EMS_EngineStatus_Convert/1 -> EMS_EngineStatus_L/1
  EMS_EngineStatus_Sub/1(Out1) -> EMS_EngineStatus_Convert/1
  EMS_EngineStatus_sat/1 -> EMS_EngineStatus_Out/1
  EMS_EngineStatus_Ad/1 -> EMS_EngineStatus_sat/1
  EMS_EngineStatus_O/1 -> EMS_EngineStatus_Ad/2
  EMS_EngineStatus_F/1 -> EMS_EngineStatus_Ad/1
  SAS_SteeringAngleValidcv/1 -> SAS_SteeringAngleValid_F/1
  SAS_SteeringAngleValid_S/1 -> SAS_SteeringAngleValidcv/1
  SAS_SteeringAngleValid_L/1 -> SAS_SteeringAngleValid_S/1
  SAS_SteeringAngleValid_Convert/1 -> SAS_SteeringAngleValid_L/1
  SAS_SteeringAngleValid_Sub/1(Out1) -> SAS_SteeringAngleValid_Convert/1
  Demux/1 -> EMS_BrakePedalStatus_Sub/1(In1), EMS_EngineStatus_Sub/1(In1), SAS_SteeringAngleValid_Sub/1(In1)
  SAS_SteeringAngleValid_sat/1 -> SAS_SteeringAngleValid_Out/1
  SAS_SteeringAngleValid_Ad/1 -> SAS_SteeringAngleValid_sat/1
  SAS_SteeringAngleValid_O/1 -> SAS_SteeringAngleValid_Ad/2
  SAS_SteeringAngleValid_F/1 -> SAS_SteeringAngleValid_Ad/1

== system VCU_CS75_12_16_Test/长安CS75底盘程序，20ms一次/Input/DBC转化的messages（存底）/ReceiveMessages22/GW_332 ==
  input : Inport
  Demux : Demux  Outputs=8
  EMS_EngineSpeed_Ad : Sum
  EMS_EngineSpeed_Convert : DataTypeConversion  OutDataTypeStr=uint32
  EMS_EngineSpeed_F : Gain  Gain=0.25
  EMS_EngineSpeed_L : simulink/Logic and Bit Operations/Bitwise Operator  logicop=AND  UseBitMask=on  BitMask=65535  BitMaskRealWorld=Stored Integer
  EMS_EngineSpeed_O : Constant  Value=0  OutDataTypeStr=single
  EMS_EngineSpeed_S : ArithShift
  EMS_EngineSpeed_Sub : Subsystem
  EMS_EngineSpeed_sat : Saturate  UpperLimit=16383.5  LowerLimit=0
  EMS_EngineSpeedcv : DataTypeConversion
  EMS_EngineSpeedinput6_Ad : Sum
  EMS_EngineSpeedinput6_C : Constant  Value=256
  EMS_EngineSpeedinput6_P : Product
  SAS_SASFailure_Ad : Sum
  SAS_SASFailure_Convert : DataTypeConversion  OutDataTypeStr=uint32
  SAS_SASFailure_F : Gain
  SAS_SASFailure_L : simulink/Logic and Bit Operations/Bitwise Operator  logicop=AND  UseBitMask=on  BitMask=16  BitMaskRealWorld=Stored Integer
  SAS_SASFailure_O : Constant  Value=0  OutDataTypeStr=single
  SAS_SASFailure_S : ArithShift  BitShiftNumber=4
  SAS_SASFailure_Sub : Subsystem
  SAS_SASFailure_sat : Saturate  UpperLimit=1  LowerLimit=0
  SAS_SASFailurecv : DataTypeConversion
  SRS_DriverBuckleSwitchStatus_Ad : Sum
  SRS_DriverBuckleSwitchStatus_Convert : DataTypeConversion  OutDataTypeStr=uint32
  SRS_DriverBuckleSwitchStatus_F : Gain
  SRS_DriverBuckleSwitchStatus_L : simulink/Logic and Bit Operations/Bitwise Operator  logicop=AND  UseBitMask=on  BitMask=192  BitMaskRealWorld=Stored Integer
  SRS_DriverBuckleSwitchStatus_O : Constant  Value=0  OutDataTypeStr=single
  SRS_DriverBuckleSwitchStatus_S : ArithShift  BitShiftNumber=6
  SRS_DriverBuckleSwitchStatus_Sub : Subsystem
  SRS_DriverBuckleSwitchStatus_sat : Saturate  UpperLimit=3  LowerLimit=0
  SRS_DriverBuckleSwitchStatuscv : DataTypeConversion
  SRS_PassengerBuckleSwitchStatus_Ad : Sum
  SRS_PassengerBuckleSwitchStatus_Convert : DataTypeConversion  OutDataTypeStr=uint32
  SRS_PassengerBuckleSwitchStatus_F : Gain
  SRS_PassengerBuckleSwitchStatus_L : simulink/Logic and Bit Operations/Bitwise Operator  logicop=AND  UseBitMask=on  BitMask=48  BitMaskRealWorld=Stored Integer
  SRS_PassengerBuckleSwitchStatus_O : Constant  Value=0  OutDataTypeStr=single
  SRS_PassengerBuckleSwitchStatus_S : ArithShift  BitShiftNumber=4
  SRS_PassengerBuckleSwitchStatus_Sub : Subsystem
  SRS_PassengerBuckleSwitchStatus_sat : Saturate  UpperLimit=3  LowerLimit=0
  SRS_PassengerBuckleSwitchStatuscv : DataTypeConversion
  SRS_PassengerBuckleSwitchStatus_Out : Outport
  SRS_DriverBuckleSwitchStatus_Out : Outport  Port=2
  SAS_SASFailure_Out : Outport  Port=3
  EMS_EngineSpeed_Out : Outport  Port=4
  wires:
  input/1 -> Demux/1
  EMS_EngineSpeedcv/1 -> EMS_EngineSpeed_F/1
  EMS_EngineSpeed_S/1 -> EMS_EngineSpeedcv/1
  EMS_EngineSpeed_L/1 -> EMS_EngineSpeed_S/1
  EMS_EngineSpeed_Convert/1 -> EMS_EngineSpeed_L/1
  EMS_EngineSpeed_Sub/1(Out1) -> EMS_EngineSpeed_Convert/1
  EMS_EngineSpeedinput6_Ad/1 -> EMS_EngineSpeed_Sub/1(In1)
  Demux/7 -> EMS_EngineSpeedinput6_Ad/2
  EMS_EngineSpeedinput6_P/1 -> EMS_EngineSpeedinput6_Ad/1
  EMS_EngineSpeedinput6_C/1 -> EMS_EngineSpeedinput6_P/2
  Demux/6 -> EMS_EngineSpeedinput6_P/1
  EMS_EngineSpeed_sat/1 -> EMS_EngineSpeed_Out/1
  EMS_EngineSpeed_Ad/1 -> EMS_EngineSpeed_sat/1
  EMS_EngineSpeed_O/1 -> EMS_EngineSpeed_Ad/2
  EMS_EngineSpeed_F/1 -> EMS_EngineSpeed_Ad/1
  SAS_SASFailurecv/1 -> SAS_SASFailure_F/1
  SAS_SASFailure_S/1 -> SAS_SASFailurecv/1
  SAS_SASFailure_L/1 -> SAS_SASFailure_S/1
  SAS_SASFailure_Convert/1 -> SAS_SASFailure_L/1
  SAS_SASFailure_Sub/1(Out1) -> SAS_SASFailure_Convert/1
  Demux/5 -> SAS_SASFailure_Sub/1(In1)
  SAS_SASFailure_sat/1 -> SAS_SASFailure_Out/1
  SAS_SASFailure_Ad/1 -> SAS_SASFailure_sat/1
  SAS_SASFailure_O/1 -> SAS_SASFailure_Ad/2
  SAS_SASFailure_F/1 -> SAS_SASFailure_Ad/1
  SRS_DriverBuckleSwitchStatuscv/1 -> SRS_DriverBuckleSwitchStatus_F/1
  SRS_DriverBuckleSwitchStatus_S/1 -> SRS_DriverBuckleSwitchStatuscv/1
  SRS_DriverBuckleSwitchStatus_L/1 -> SRS_DriverBuckleSwitchStatus_S/1
  SRS_DriverBuckleSwitchStatus_Convert/1 -> SRS_DriverBuckleSwitchStatus_L/1
  SRS_DriverBuckleSwitchStatus_Sub/1(Out1) -> SRS_DriverBuckleSwitchStatus_Convert/1
  SRS_DriverBuckleSwitchStatus_sat/1 -> SRS_DriverBuckleSwitchStatus_Out/1
  SRS_DriverBuckleSwitchStatus_Ad/1 -> SRS_DriverBuckleSwitchStatus_sat/1
  SRS_DriverBuckleSwitchStatus_O/1 -> SRS_DriverBuckleSwitchStatus_Ad/2
  SRS_DriverBuckleSwitchStatus_F/1 -> SRS_DriverBuckleSwitchStatus_Ad/1
  SRS_PassengerBuckleSwitchStatuscv/1 -> SRS_PassengerBuckleSwitchStatus_F/1
  SRS_PassengerBuckleSwitchStatus_S/1 -> SRS_PassengerBuckleSwitchStatuscv/1
  SRS_PassengerBuckleSwitchStatus_L/1 -> SRS_PassengerBuckleSwitchStatus_S/1
  SRS_PassengerBuckleSwitchStatus_Convert/1 -> SRS_PassengerBuckleSwitchStatus_L/1
  SRS_PassengerBuckleSwitchStatus_Sub/1(Out1) -> SRS_PassengerBuckleSwitchStatus_Convert/1
  Demux/4 -> SRS_DriverBuckleSwitchStatus_Sub/1(In1), SRS_PassengerBuckleSwitchStatus_Sub/1(In1)
  SRS_PassengerBuckleSwitchStatus_sat/1 -> SRS_PassengerBuckleSwitchStatus_Out/1
  SRS_PassengerBuckleSwitchStatus_Ad/1 -> SRS_PassengerBuckleSwitchStatus_sat/1
  SRS_PassengerBuckleSwitchStatus_O/1 -> SRS_PassengerBuckleSwitchStatus_Ad/2
  SRS_PassengerBuckleSwitchStatus_F/1 -> SRS_PassengerBuckleSwitchStatus_Ad/1

== system VCU_CS75_12_16_Test/长安CS75底盘程序，20ms一次/Input/DBC转化的messages（存底）/ReceiveMessages23/GW_308 ==
  input : Inport
  Demux : Demux  Outputs=8
  IP_TotalOdometer_Ad : Sum
  IP_TotalOdometer_Convert : DataTypeConversion  OutDataTypeStr=uint32
  IP_TotalOdometer_F : Gain  Gain=0.1
  IP_TotalOdometer_L : simulink/Logic and Bit Operations/Bitwise Operator  logicop=AND  UseBitMask=on  BitMask=16777215  BitMaskRealWorld=Stored Integer
  IP_TotalOdometer_O : Constant  Value=0  OutDataTypeStr=single
  IP_TotalOdometer_S : ArithShift
  IP_TotalOdometer_Sub : Subsystem
  IP_TotalOdometer_sat : Saturate  UpperLimit=999999  LowerLimit=0
  IP_TotalOdometercv : DataTypeConversion
  IP_TotalOdometerinput5_Ad : Sum
  IP_TotalOdometerinput5_C : Constant  Value=65536
  IP_TotalOdometerinput5_P : Product
  IP_TotalOdometerinput6_Ad : Sum
  IP_TotalOdometerinput6_C : Constant  Value=256
  IP_TotalOdometerinput6_P : Product
  IP_TotalOdometer_Out : Outport
  wires:
  input/1 -> Demux/1
  IP_TotalOdometercv/1 -> IP_TotalOdometer_F/1
  IP_TotalOdometer_S/1 -> IP_TotalOdometercv/1
  IP_TotalOdometer_L/1 -> IP_TotalOdometer_S/1
  IP_TotalOdometer_Convert/1 -> IP_TotalOdometer_L/1
  IP_TotalOdometer_Sub/1(Out1) -> IP_TotalOdometer_Convert/1
  IP_TotalOdometerinput6_Ad/1 -> IP_TotalOdometer_Sub/1(In1)
  IP_TotalOdometerinput5_Ad/1 -> IP_TotalOdometerinput6_Ad/2
  IP_TotalOdometerinput6_P/1 -> IP_TotalOdometerinput6_Ad/1
  IP_TotalOdometerinput6_C/1 -> IP_TotalOdometerinput6_P/2
  Demux/6 -> IP_TotalOdometerinput6_P/1
  Demux/7 -> IP_TotalOdometerinput5_Ad/2
  IP_TotalOdometerinput5_P/1 -> IP_TotalOdometerinput5_Ad/1
  IP_TotalOdometerinput5_C/1 -> IP_TotalOdometerinput5_P/2
  Demux/5 -> IP_TotalOdometerinput5_P/1
  IP_TotalOdometer_sat/1 -> IP_TotalOdometer_Out/1
  IP_TotalOdometer_Ad/1 -> IP_TotalOdometer_sat/1
  IP_TotalOdometer_O/1 -> IP_TotalOdometer_Ad/2
  IP_TotalOdometer_F/1 -> IP_TotalOdometer_Ad/1

== system VCU_CS75_12_16_Test/长安CS75底盘程序，20ms一次/Input/DBC转化的messages（存底）/ReceiveMessages24/GW_376 ==
  input : Inport
  Demux : Demux  Outputs=8
  EMS_ConditionIdle_Ad : Sum
  EMS_ConditionIdle_Convert : DataTypeConversion  OutDataTypeStr=uint32
  EMS_ConditionIdle_F : Gain
  EMS_ConditionIdle_L : simulink/Logic and Bit Operations/Bitwise Operator  logicop=AND  UseBitMask=on  BitMask=128  BitMaskRealWorld=Stored Integer
  EMS_ConditionIdle_O : Constant  Value=0  OutDataTypeStr=single
  EMS_ConditionIdle_S : ArithShift  BitShiftNumber=7
  EMS_ConditionIdle_Sub : Subsystem
  EMS_ConditionIdle_sat : Saturate  UpperLimit=1  LowerLimit=0
  EMS_ConditionIdlecv : DataTypeConversion
  EMS_EngineFuelCutOff_Ad : Sum
  EMS_EngineFuelCutOff_Convert : DataTypeConversion  OutDataTypeStr=uint32
  EMS_EngineFuelCutOff_F : Gain
  EMS_EngineFuelCutOff_L : simulink/Logic and Bit Operations/Bitwise Operator  logicop=AND  UseBitMask=on  BitMask=16  BitMaskRealWorld=Stored Integer
  EMS_EngineFuelCutOff_O : Constant  Value=0  OutDataTypeStr=single
  EMS_EngineFuelCutOff_S : ArithShift  BitShiftNumber=4
  EMS_EngineFuelCutOff_Sub : Subsystem
  EMS_EngineFuelCutOff_sat : Saturate  UpperLimit=1  LowerLimit=0
  EMS_EngineFuelCutOffcv : DataTypeConversion
  EMS_FrictionalTorq_Ad : Sum
  EMS_FrictionalTorq_Convert : DataTypeConversion  OutDataTypeStr=uint32
  EMS_FrictionalTorq_F : Gain  Gain=0.001526
  EMS_FrictionalTorq_L : simulink/Logic and Bit Operations/Bitwise Operator  logicop=AND  UseBitMask=on  BitMask=65535  BitMaskRealWorld=Stored Integer
  EMS_FrictionalTorq_O : Constant  Value=0  OutDataTypeStr=single
  EMS_FrictionalTorq_S : ArithShift
  EMS_FrictionalTorq_Sub : Subsystem
  EMS_FrictionalTorq_sat : Saturate  UpperLimit=3000  LowerLimit=0
  EMS_FrictionalTorqcv : DataTypeConversion
  EMS_FrictionalTorqinput2_Ad : Sum
  EMS_FrictionalTorqinput2_C : Constant  Value=256
  EMS_FrictionalTorqinput2_P : Product
  EMS_TorqueConstant_Ad : Sum
  EMS_TorqueConstant_Convert : DataTypeConversion  OutDataTypeStr=uint32
  EMS_TorqueConstant_F : Gain  Gain=10
  EMS_TorqueConstant_L : simulink/Logic and Bit Operations/Bitwise Operator  logicop=AND  UseBitMask=on  BitMask=255  BitMaskRealWorld=Stored Integer
  EMS_TorqueConstant_O : Constant  Value=0  OutDataTypeStr=single
  EMS_TorqueConstant_S : ArithShift
  EMS_TorqueConstant_Sub : Subsystem
  EMS_TorqueConstant_sat : Saturate  UpperLimit=2540  LowerLimit=0
  EMS_TorqueConstantcv : DataTypeConversion
  EMS_TorqueConstant_Out : Outport
  EMS_FrictionalTorq_Out : Outport  Port=2
  EMS_EngineFuelCutOff_Out : Outport  Port=3
  EMS_ConditionIdle_Out : Outport  Port=4
  wires:
  input/1 -> Demux/1
  EMS_ConditionIdlecv/1 -> EMS_ConditionIdle_F/1
  EMS_ConditionIdle_S/1 -> EMS_ConditionIdlecv/1
  EMS_ConditionIdle_L/1 -> EMS_ConditionIdle_S/1
  EMS_ConditionIdle_Convert/1 -> EMS_ConditionIdle_L/1
  EMS_ConditionIdle_Sub/1(Out1) -> EMS_ConditionIdle_Convert/1
  EMS_ConditionIdle_sat/1 -> EMS_ConditionIdle_Out/1
  EMS_ConditionIdle_Ad/1 -> EMS_ConditionIdle_sat/1
  EMS_ConditionIdle_O/1 -> EMS_ConditionIdle_Ad/2
  EMS_ConditionIdle_F/1 -> EMS_ConditionIdle_Ad/1
  EMS_EngineFuelCutOffcv/1 -> EMS_EngineFuelCutOff_F/1
  EMS_EngineFuelCutOff_S/1 -> EMS_EngineFuelCutOffcv/1
  EMS_EngineFuelCutOff_L/1 -> EMS_EngineFuelCutOff_S/1
  EMS_EngineFuelCutOff_Convert/1 -> EMS_EngineFuelCutOff_L/1
  EMS_EngineFuelCutOff_Sub/1(Out1) -> EMS_EngineFuelCutOff_Convert/1
  Demux/4 -> EMS_ConditionIdle_Sub/1(In1), EMS_EngineFuelCutOff_Sub/1(In1)
  EMS_EngineFuelCutOff_sat/1 -> EMS_EngineFuelCutOff_Out/1
  EMS_EngineFuelCutOff_Ad/1 -> EMS_EngineFuelCutOff_sat/1
  EMS_EngineFuelCutOff_O/1 -> EMS_EngineFuelCutOff_Ad/2
  EMS_EngineFuelCutOff_F/1 -> EMS_EngineFuelCutOff_Ad/1
  EMS_FrictionalTorqcv/1 -> EMS_FrictionalTorq_F/1
  EMS_FrictionalTorq_S/1 -> EMS_FrictionalTorqcv/1
  EMS_FrictionalTorq_L/1 -> EMS_FrictionalTorq_S/1
  EMS_FrictionalTorq_Convert/1 -> EMS_FrictionalTorq_L/1
  EMS_FrictionalTorq_Sub/1(Out1) -> EMS_FrictionalTorq_Convert/1
  EMS_FrictionalTorqinput2_Ad/1 -> EMS_FrictionalTorq_Sub/1(In1)
  Demux/3 -> EMS_FrictionalTorqinput2_Ad/2
  EMS_FrictionalTorqinput2_P/1 -> EMS_FrictionalTorqinput2_Ad/1
  EMS_FrictionalTorqinput2_C/1 -> EMS_FrictionalTorqinput2_P/2
  Demux/2 -> EMS_FrictionalTorqinput2_P/1
  EMS_FrictionalTorq_sat/1 -> EMS_FrictionalTorq_Out/1
  EMS_FrictionalTorq_Ad/1 -> EMS_FrictionalTorq_sat/1
  EMS_FrictionalTorq_O/1 -> EMS_FrictionalTorq_Ad/2
  EMS_FrictionalTorq_F/1 -> EMS_FrictionalTorq_Ad/1
  EMS_TorqueConstantcv/1 -> EMS_TorqueConstant_F/1
  EMS_TorqueConstant_S/1 -> EMS_TorqueConstantcv/1
  EMS_TorqueConstant_L/1 -> EMS_TorqueConstant_S/1
  EMS_TorqueConstant_Convert/1 -> EMS_TorqueConstant_L/1
  EMS_TorqueConstant_Sub/1(Out1) -> EMS_TorqueConstant_Convert/1
  Demux/1 -> EMS_TorqueConstant_Sub/1(In1)
  EMS_TorqueConstant_sat/1 -> EMS_TorqueConstant_Out/1
  EMS_TorqueConstant_Ad/1 -> EMS_TorqueConstant_sat/1
  EMS_TorqueConstant_O/1 -> EMS_TorqueConstant_Ad/2
  EMS_TorqueConstant_F/1 -> EMS_TorqueConstant_Ad/1
